simulink model "Rail_SetPointAddCor"  (R2016b)
settings: configuration reference "CodeGenConfigSet" (kept outside this file)
values from neighbouring files (symbols this model uses):
  Rail_facSetPointFTSCor_CUR = Calibration.Parameter    [init_Rail_SetPointAddCor.m]
  Rail_facSetPointFTSCor_CURX = Calibration.Parameter    [init_Rail_SetPointAddCor.m]
  Rail_pSetPointFTSCor_MAP = Calibration.Parameter    [init_Rail_SetPointAddCor.m]
  Rail_pSetPointFTSCor_MAPX = Calibration.Parameter    [init_Rail_SetPointAddCor.m]
  Rail_pSetPointFTSCor_MAPY = Calibration.Parameter    [init_Rail_SetPointAddCor.m]
  Rail_pSetPointMax_MAP = Calibration.Parameter    [init_Rail_SetPointAddCor.m]
  Rail_pSetPointMax_MAPX = Calibration.Parameter    [init_Rail_SetPointAddCor.m]
  Rail_pSetPointMax_MAPY = Calibration.Parameter    [init_Rail_SetPointAddCor.m]
  Rail_pSetPointMaxDef_C = Calibration.Parameter    [init_Rail_SetPointAddCor.m]
  Rail_pSetPointMin_MAP = Calibration.Parameter    [init_Rail_SetPointAddCor.m]
  Rail_pSetPointMin_MAPX = Calibration.Parameter    [init_Rail_SetPointAddCor.m]
  Rail_pSetPointMin_MAPY = Calibration.Parameter    [init_Rail_SetPointAddCor.m]
  Rail_pSetPointMinDef_C = Calibration.Parameter    [init_Rail_SetPointAddCor.m]
  Rail_pSetPointTolcMin_C = Calibration.Parameter    [init_Rail_SetPointAddCor.m]
undefined symbols (not defined in the file or in its folder): RailCtl_State_conv
settings Model: Creator=lenovo  LastModifiedBy=mayongchao
settings ConfigSetRef: SourceLocation=Base Workspace

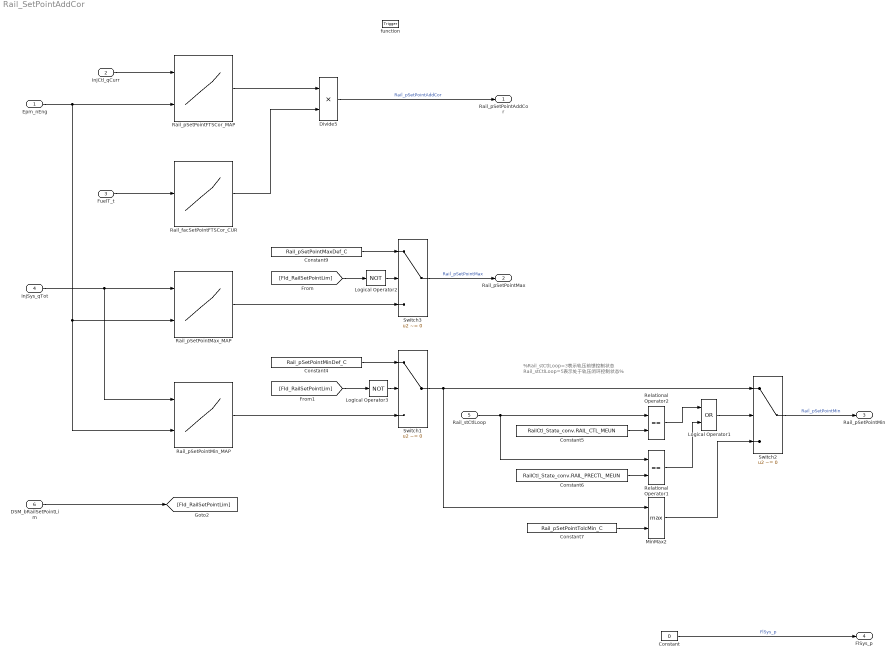
== system Rail_SetPointAddCor ==
  note: %Rail_stCtlLoop=3表示轨压前馈控制状态
      | Rail_stCtlLoop=5表示处于轨压闭环控制状态%
  Epm_nEng : Inport  Tag=rpm  Description=Engine speed  OutMin=0  OutMax=6000  OutDataTypeStr=EngSpeed_rpm
  InjCtl_qCurr : Inport  Tag=mg/hub  Description=Torque generating engine fuel injection quantity  Port=2  OutMin=-319  OutMax=319  OutDataTypeStr=FuelMass_mg_hub
  FuelT_t : Inport  Tag=deg  Description=Temperature of fuel  Port=3  OutMin=-50  OutMax=150  OutDataTypeStr=Temp_deg
  InjSys_qTot : Inport  Tag=mg/hub  Description=Total engine injection quantity  Port=4  OutMin=-319  OutMax=319  OutDataTypeStr=FuelMass_mg_hub
  Rail_stCtlLoop : Inport  Description=State of the rail pressure governor control  Port=5  OutDataTypeStr=Enum: RailCtl_State_conv
  DSM_bRailSetPointLim : Inport  Description=state of FId_RailSetPointLim  Port=6  OutMin=0  OutMax=1  OutDataTypeStr=boolean
  function : TriggerPort  TriggerType=function-call  VariantControl=Variant
  Constant : Constant  Value=0  OutDataTypeStr=Inherit: Inherit via back propagation  SampleTime=-1
  Constant4 : Constant  Value=Rail_pSetPointMinDef_C  SampleTime=-1
  Constant5 : Constant  Value=RailCtl_State_conv.RAIL_CTL_MEUN  OutDataTypeStr=Inherit: Inherit via back propagation  SampleTime=-1
  Constant6 : Constant  Value=RailCtl_State_conv.RAIL_PRECTL_MEUN  OutDataTypeStr=Inherit: Inherit via back propagation
  Constant7 : Constant  Value=Rail_pSetPointTolcMin_C  SampleTime=-1
  Constant9 : Constant  Value=Rail_pSetPointMaxDef_C  SampleTime=-1
  Divide5 : Product  Inputs=**  OutDataTypeStr=RailPressure_bar  SaturateOnIntegerOverflow=on
  Logical Operator1 : Logic  Operator=OR  AllPortsSameDT=off  OutDataTypeStr=boolean
  Logical Operator2 : Logic  Operator=NOT  Inputs=1  AllPortsSameDT=off  OutDataTypeStr=boolean
  Logical Operator3 : Logic  Operator=NOT  Inputs=1  AllPortsSameDT=off  OutDataTypeStr=boolean
  MinMax2 : MinMax  Function=max  Inputs=2  InputSameDT=on
  Rail_facSetPointFTSCor_CUR : Lookup_n-D  NumberOfTableDimensions=1  BreakpointsForDimension1=Rail_facSetPointFTSCor_CURX  IndexSearchMethod=Linear search  BeginIndexSearchUsingPreviousIndexResult=on  Table=Rail_facSetPointFTSCor_CUR  ExtrapMethod=Clip  UseLastTableValue=on  InternalRulePriority=Speed  OutDataTypeStr=Inherit: Inherit via back propagation  SaturateOnIntegerOverflow=on
  Rail_pSetPointFTSCor_MAP : Lookup_n-D  BreakpointsForDimension1=Rail_pSetPointFTSCor_MAPY  BreakpointsForDimension2=Rail_pSetPointFTSCor_MAPX  IndexSearchMethod=Linear search  BeginIndexSearchUsingPreviousIndexResult=on  Table=Rail_pSetPointFTSCor_MAP  ExtrapMethod=Clip  UseLastTableValue=on  InternalRulePriority=Speed  OutDataTypeStr=Inherit: Inherit via back propagation  SaturateOnIntegerOverflow=on
  Rail_pSetPointMax_MAP : Lookup_n-D  BreakpointsForDimension1=Rail_pSetPointMax_MAPY  BreakpointsForDimension2=Rail_pSetPointMax_MAPX  IndexSearchMethod=Linear search  BeginIndexSearchUsingPreviousIndexResult=on  Table=Rail_pSetPointMax_MAP  ExtrapMethod=Clip  UseLastTableValue=on  InternalRulePriority=Speed  OutDataTypeStr=Inherit: Inherit via back propagation  SaturateOnIntegerOverflow=on
  Rail_pSetPointMin_MAP : Lookup_n-D  BreakpointsForDimension1=Rail_pSetPointMin_MAPY  BreakpointsForDimension2=Rail_pSetPointMin_MAPX  IndexSearchMethod=Linear search  BeginIndexSearchUsingPreviousIndexResult=on  Table=Rail_pSetPointMin_MAP  ExtrapMethod=Clip  UseLastTableValue=on  InternalRulePriority=Speed  OutDataTypeStr=Inherit: Inherit via back propagation  SaturateOnIntegerOverflow=on
  Relational Operator1 : RelationalOperator  Operator===  OutDataTypeStr=boolean  RndMeth=Nearest  InputSameDT=on
  Relational Operator2 : RelationalOperator  Operator===  OutDataTypeStr=boolean  RndMeth=Nearest  InputSameDT=on
  Switch1 : Switch  Criteria=u2 ~= 0  InputSameDT=on
  Switch2 : Switch  Criteria=u2 ~= 0  InputSameDT=on
  Switch3 : Switch  Criteria=u2 ~= 0  InputSameDT=on
  Rail_pSetPointAddCor : Outport  Tag=bar  Description=Buffer variable for additional correction rail setpoint values which were received via the remote function Rail_SetPointAddCor.  OutMin=-2500  OutMax=2500  OutDataTypeStr=RailPressure_bar
  Rail_pSetPointMax : Outport  Tag=bar  Description=Maximum rail pressure setpoint  Port=2  OutMin=-2500  OutMax=2500  OutDataTypeStr=RailPressure_bar
  Rail_pSetPointMin : Outport  Tag=bar  Description=Minimum rail pressure setpoint  Port=3  OutMin=-2500  OutMax=2500  OutDataTypeStr=RailPressure_bar
  FlSys_p : Outport  Tag=kPa  Description=Fuelpressure on high pressure pump  Port=4  OutMin=0  OutMax=3000  OutDataTypeStr=AirPressure_kPa
  wires:
  DSM_bRailSetPointLim/1 -> [FId_RailSetPointLim]
  InjCtl_qCurr/1 -> Rail_pSetPointFTSCor_MAP/1
  Rail_pSetPointMax_MAP/1 -> Switch3/3
  Rail_facSetPointFTSCor_CUR/1 -> Divide5/2
  Rail_pSetPointFTSCor_MAP/1 -> Divide5/1
  Constant5/1 -> Relational Operator2/2
  Constant4/1 -> Switch1/1
  Constant7/1 -> MinMax2/2
  Switch1/1 -> MinMax2/1, Switch2/1
  Switch3/1 -> Rail_pSetPointMax/1  "Rail_pSetPointMax"
  InjSys_qTot/1 -> Rail_pSetPointMax_MAP/1, Rail_pSetPointMin_MAP/1
  [FId_RailSetPointLim] -> Logical Operator3/1
  Rail_stCtlLoop/1 -> Relational Operator1/1, Relational Operator2/1
  Logical Operator1/1 -> Switch2/2
  [FId_RailSetPointLim] -> Logical Operator2/1
  Divide5/1 -> Rail_pSetPointAddCor/1  "Rail_pSetPointAddCor"
  Switch2/1 -> Rail_pSetPointMin/1  "Rail_pSetPointMin"
  Epm_nEng/1 -> Rail_pSetPointMax_MAP/2, Rail_pSetPointMin_MAP/2, Rail_pSetPointFTSCor_MAP/2
  Rail_pSetPointMin_MAP/1 -> Switch1/3
  Constant6/1 -> Relational Operator1/2
  Constant9/1 -> Switch3/1
  FuelT_t/1 -> Rail_facSetPointFTSCor_CUR/1
  Relational Operator2/1 -> Logical Operator1/1
  Relational Operator1/1 -> Logical Operator1/2
  MinMax2/1 -> Switch2/3
  Logical Operator2/1 -> Switch3/2
  Logical Operator3/1 -> Switch1/2
  Constant/1 -> FlSys_p/1  "FlSys_p"
